simulink model "cv5_model"  (R2019b)
settings: Solver=FixedStepAuto  StartTime=0.0  StopTime=1040  FixedStep=1  RelTol=1e-3
values from neighbouring files (symbols this model uses):
  AG = 0.95    [identifikacia_simulatora.m]    (also in identifikacia_simulatora2.m; simulator.m)
  G_b = 8.5    [cv5.m]    (also in identifikacia_simulatora.m = 8.8; identifikacia_simulatora2.m; simulator.m)
  G_INIT = 153    [cv5.m]    (also in identifikacia_simulatora.m = 158.4; identifikacia_simulatora2.m; simulator.m)
  IB_INIT = 6.5    [identifikacia_simulatora.m]    (also in identifikacia_simulatora2.m; simulator.m)
  ki = 0.1645    [cv5.m]    (also in identifikacia_simulatora.m; identifikacia_simulatora2.m = 0.1939; simulator.m)
  p2 = 0.0106    [cv5.m]    (also in identifikacia_simulatora.m; identifikacia_simulatora2.m = 0.0097; simulator.m)
  S_G = 0    [cv5.m]    (also in identifikacia_simulatora.m = 0.032; simulator.m = 0.032)
  SI = S_I    (= 0.00159)    [identifikacia_simulatora.m]    (also in identifikacia_simulatora2.m = 0.0014; simulator.m)
  TD = 33.474    [identifikacia_simulatora.m]    (also in identifikacia_simulatora2.m = 41.1727; simulator.m)
  TI = 44.55    [cv5.m]    (also in identifikacia_simulatora.m; identifikacia_simulatora2.m = 42.8216; simulator.m)
  V_G = 1.467    [cv5.m]    (also in identifikacia_simulatora.m; identifikacia_simulatora2.m; simulator.m)
  VI = 138.8    [cv5.m]    (also in identifikacia_simulatora.m; identifikacia_simulatora2.m = 110.599; simulator.m)
undefined symbols (not defined in the file or in its folder): sigbuilder_block
settings Model: Creator=kaspe  LastModifiedBy=shneeder
settings DataIOCC: ReturnWorkspaceOutputs=off
settings DebuggingCC: ArithmeticOperatorsInVariantConditions=warning
settings SFSimCC: CustomCodeUndefinedFunction=UseInterfaceOnly

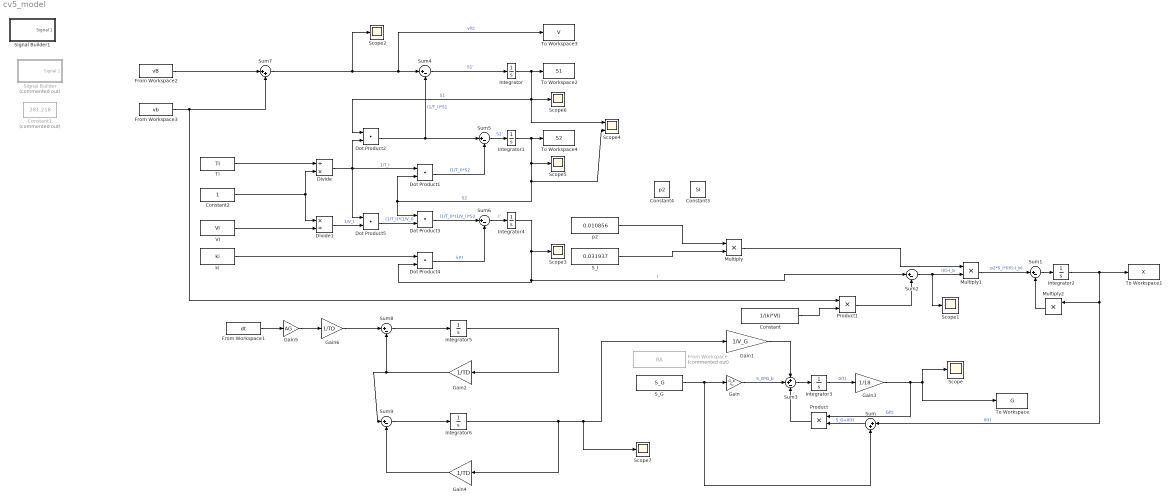
== system cv5_model ==
  Constant : Constant  Value=1/(ki*VI)
  Constant1 : Constant  Commented=on  Value=281.218
  Constant2 : Constant
  Constant3 : Constant  Value=SI
  Constant4 : Constant  Value=p2
  Divide : Product  Inputs=/*
  Divide1 : Product  Inputs=*/
  Dot Product{1..5} (5 alike) : DotProduct  InputSameDT=on  OutDataTypeStr=Inherit: Inherit via internal rule
  From Workspace : FromWorkspace  Commented=on  VariableName=RA  SampleTime=0
  From Workspace1 : FromWorkspace  VariableName=dt  SampleTime=0
  From Workspace2 : FromWorkspace  VariableName=vB  SampleTime=0
  From Workspace3 : FromWorkspace  VariableName=vb  SampleTime=0
  Gain : Gain  Gain=G_b  Multiplication=Matrix(K*u)
  Gain1 : Gain  Gain=1/V_G
  Gain2 : Gain  Gain=1/TD
  Gain3 : Gain  Gain=1/18
  Gain4 : Gain  Gain=1/TD
  Gain5 : Gain  Gain=AG
  Gain6 : Gain  Gain=1/TD
  Integrator{,1..2,5..6} (5 alike) : Integrator
  Integrator3 : Integrator  InitialCondition=G_INIT
  Integrator4 : Integrator  InitialCondition=IB_INIT
  Multiply : Product
  Multiply1 : Product
  Multiply2 : Product
  Product : Product
  Product1 : Product
  S_G : Constant  Value=S_G
  S_I : Constant  Value=0.031937
  Scope{,1..3,5..7} (7 alike) : Scope
  Scope4 : Scope  NumInputPorts=2
  Signal Builder : Subsystem  Tag=STV Subsys  Commented=on  LoadFcn=sigbuilder_block('load');  StartFcn=sigbuilder_block('start');  StopFcn=sigbuilder_block('stop');  ClipboardFcn=sigbuilder_block('clipboard');  mask(Sigbuilder block){tuvar=[0:10]}
      mask help: Simulink:masks:SigbuilderBlock_MD
      mask init:
      | if ~strcmp(get_param(bdroot(gcbh),'SimulationStatus'),'stopped') tuvar = sigbuilder_block('maskInit'); end
      settings: CopyFcn=sigbuilder_block('copy');  DeleteFcn=sigbuilder_block('delete');  ModelCloseFcn=sigbuilder_block('modelClose');  PreSaveFcn=sigbuilder_block('preSave');  PauseFcn=sigbuilder_block('pause');  ContinueFcn=sigbuilder_block('continue');  NameChangeFcn=sigbuilder_block('namechange');  OpenFcn=sigbuilder_block('open',[54 30 1141.5 522.6 ]);  CloseFcn=sigbuilder_block('close');
      mask Display: plot(0, 0, 100, 100,[2, 2, 32, 32, 2], [68, 8, 8, 68, 68],[32, 2], [38, 38], [32, 19, 2],[53, 60, 44], [32, 17, 17, 2],[16, 16, 31, 31]);txt = getActiveGroup(gcbh);text(2, 100, txt,'verticalAlignment', 'top');
  Signal Builder1 : Subsystem  Tag=STV Subsys  LoadFcn=sigbuilder_block('load');  StartFcn=sigbuilder_block('start');  StopFcn=sigbuilder_block('stop');  ClipboardFcn=sigbuilder_block('clipboard');  mask(Sigbuilder block){tuvar=[0:10]}
      mask help: Simulink:masks:SigbuilderBlock_MD
      mask init:
      | if ~strcmp(get_param(bdroot(gcbh),'SimulationStatus'),'stopped') tuvar = sigbuilder_block('maskInit'); end
      settings: CopyFcn=sigbuilder_block('copy');  DeleteFcn=sigbuilder_block('delete');  ModelCloseFcn=sigbuilder_block('modelClose');  PreSaveFcn=sigbuilder_block('preSave');  PauseFcn=sigbuilder_block('pause');  ContinueFcn=sigbuilder_block('continue');  NameChangeFcn=sigbuilder_block('namechange');  OpenFcn=sigbuilder_block('open',[437.6 199.2 550.4 400 ]);  CloseFcn=sigbuilder_block('close');
      mask Display: plot(0, 0, 100, 100,[2, 2, 32, 32, 2], [68, 8, 8, 68, 68],[32, 2], [38, 38], [32, 19, 2],[53, 60, 44], [32, 17, 17, 2],[16, 16, 31, 31]);txt = getActiveGroup(gcbh);text(2, 100, txt,'verticalAlignment', 'top');
  Sum : Sum  Inputs=|++
  Sum{1..2,4..6,8..9} (7 alike) : Sum  Inputs=|+-
  Sum3 : Sum  Inputs=++-
  Sum7 : Sum  Inputs=|++
  TI : Constant  Value=TI
  To Workspace : ToWorkspace  VariableName=G  SaveFormat=Timeseries  SampleTime=-1
  To Workspace1 : ToWorkspace  VariableName=X  SaveFormat=Timeseries  SampleTime=-1
  To Workspace2 : ToWorkspace  VariableName=S1  SaveFormat=Timeseries  SampleTime=-1
  To Workspace3 : ToWorkspace  VariableName=V  SaveFormat=Timeseries  SampleTime=-1
  To Workspace4 : ToWorkspace  VariableName=S2  SaveFormat=Timeseries  SampleTime=-1
  VI : Constant  Value=VI
  ki : Constant  Value=ki
  p2 : Constant  Value=0.010856
  wires:
  S_G/1 -> Sum/2, Gain/1
  Sum/1 -> Product/2  "S_G+X(t)"
  Product1/1 -> Sum2/2
  Gain3/1 -> To Workspace/1, Scope/1, Product/1  "G(t)"
  Multiply/1 -> Multiply1/1
  Multiply2/1 -> Sum1/2
  Sum1/1 -> Integrator2/1
  Integrator2/1 -> To Workspace1/1, Sum/1, Multiply2/1  "X(t)"
  Gain/1 -> Sum3/2  "S_G*G_b"
  Product/1 -> Sum3/3
  Sum2/1 -> Scope1/1, Multiply1/2  "I(t)-I_b"
  Multiply1/1 -> Sum1/1  "p2*S_I*(I(t)-I_b)"
  Sum3/1 -> Integrator3/1
  Constant2/1 -> Divide1/1, Divide/2
  Integrator/1 -> Dot Product2/1, Scope4/1, Scope6/1, To Workspace2/1  "S1"
  Dot Product4/1 -> Sum6/2  "ki*I"
  Dot Product5/1 -> Dot Product3/2  "(1/T_I)*(1/V_I)"
  Dot Product3/1 -> Sum6/1  "(1/T_I)*(1/V_I)*S2"
  Sum7/1 -> To Workspace3/1, Sum4/1, Scope2/1  "v(t)"
  Dot Product1/1 -> Sum5/2  "(1/T_I)*S2"
  Divide1/1 -> Dot Product5/2  "1/V_I"
  Sum5/1 -> Integrator1/1  "S2'"
  Sum6/1 -> Integrator4/1  "I'"
  Integrator4/1 -> Sum2/1, Dot Product4/2, Scope3/1  "I"
  Sum4/1 -> Integrator/1  "S1'"
  Divide/1 -> Dot Product1/1, Dot Product2/2, Dot Product5/1  "1/T_I"
  Dot Product2/1 -> Sum5/1, Sum4/2  "(1/T_I)*S1"
  VI/1 -> Divide1/2
  TI/1 -> Divide/1
  ki/1 -> Dot Product4/1
  Integrator1/1 -> Dot Product3/1, Dot Product1/2, Scope4/2, Scope5/1, To Workspace4/1  "S2"
  Gain1/1 -> Sum3/1
  Sum9/1 -> Integrator6/1
  Sum8/1 -> Integrator5/1
  Integrator5/1 -> Gain2/1
  Integrator6/1 -> Gain4/1, Scope7/1, Gain1/1
  Gain2/1 -> Sum8/2, Sum9/1
  Gain4/1 -> Sum9/2
  From Workspace1/1 -> Gain5/1
  Gain5/1 -> Gain6/1
  Gain6/1 -> Sum8/1
  From Workspace3/1 -> Product1/1, Sum7/2
  From Workspace2/1 -> Sum7/1
  Constant/1 -> Product1/2
  Integrator3/1 -> Gain3/1  "G(t)"
  S_I/1 -> Multiply/2
  p2/1 -> Multiply/1

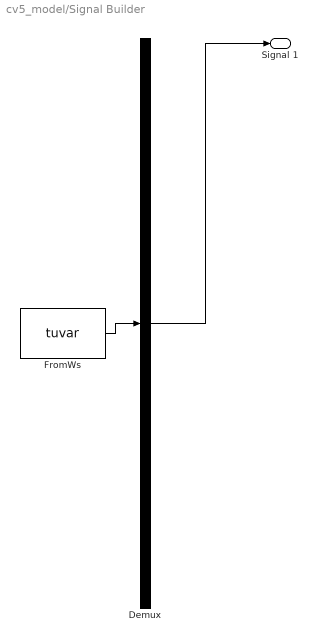
== system cv5_model/Signal Builder ==
  Demux : Demux  Tag=STV Demux  Outputs=1
  FromWs : FromWorkspace  Tag=STV FromWs  VariableName=tuvar  SampleTime=0
      SigBuilderData=|
      | common.afterFinalStr = 'Extrapolate'
      | common.sampleTime = 0
      | dataSet.timeRange = [0 599]
      | dataSet.name = 'Group 1'
      | sbobj.Groups.Name = 'Group 1'
      | sbobj.Groups.Signals.Name = 'Signal 1'
      | sbobj.Groups.Signals.XData = [0 5 5 599]
      | sbobj.Groups.Signals.YData = [40000 40000 0 0]
      | sbobj.Groups.TimeRange = [0 599]
  Signal 1 : Outport  Tag=STV Outport  VectorParamsAs1DForOutWhenUnconnected=off
  wires:
  Demux/1 -> Signal 1/1
  FromWs/1 -> Demux/1

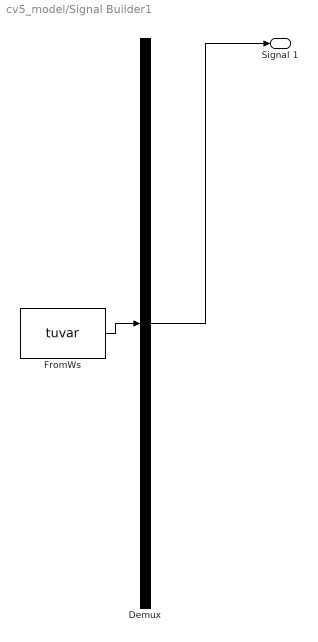
== system cv5_model/Signal Builder1 ==
  Demux : Demux  Tag=STV Demux  Outputs=1
  FromWs : FromWorkspace  Tag=STV FromWs  VariableName=tuvar  SampleTime=0
      SigBuilderData=|
      | common.afterFinalStr = 'Extrapolate'
      | common.sampleTime = 0
      | dataSet.timeRange = [0 1440]
      | dataSet.name = 'Group 1'
      | sbobj.Groups.Name = 'Group 1'
      | sbobj.Groups.Signals.Name = 'Signal 1'
      | sbobj.Groups.Signals.XData = [0 4 6 496 496 499 1440]
      | sbobj.Groups.Signals.YData = [0 0 0 0 129500 0 0]
      | sbobj.Groups.TimeRange = [0 1440]
  Signal 1 : Outport  Tag=STV Outport
  wires:
  Demux/1 -> Signal 1/1
  FromWs/1 -> Demux/1
